simulink model "Drone_simulation_pilotage_en_vitesse_v5"  (R2016a)
settings: Solver=ode15s  StartTime=0.0  StopTime=6  FixedStep=0.01  MaxStep=0.01  RelTol=1e-3
undefined symbols (not defined in the file or in its folder): faut_sldprt, sigbuilder_block, sol_D, X, Y, Z
libraries: fl_lib x78, sm_lib x36, nesl_utility x15, simulink x1
(part 2 of 2)

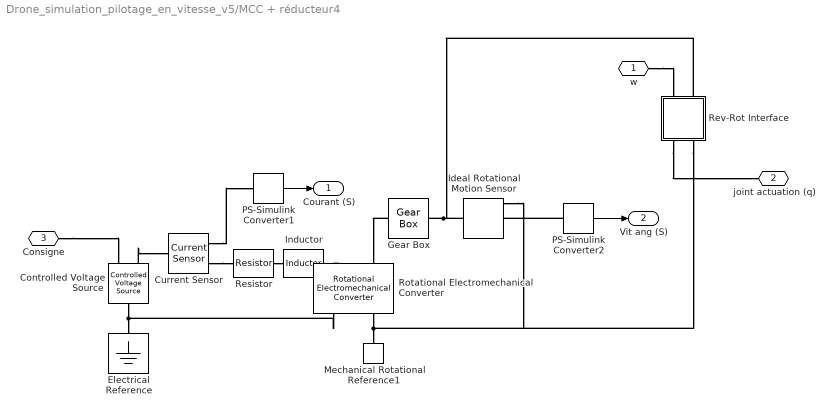
== system Drone_simulation_pilotage_en_vitesse_v5/MCC + réducteur4 ==
  Controlled Voltage Source : fl_lib/Electrical/Electrical Sources/Controlled Voltage Source
  Current Sensor : fl_lib/Electrical/Electrical Sensors/Current Sensor
  Electrical Reference : fl_lib/Electrical/Electrical Elements/Electrical Reference
  Gear Box : fl_lib/Mechanical/Mechanisms/Gear Box  ratio=6  t_in_specify=off  t_in_priority=High  t_in=0 N*m  t_out_specify=off  t_out_priority=High  t_out=0 N*m
  Ideal Rotational Motion Sensor : fl_lib/Mechanical/Mechanical Sensors/Ideal Rotational Motion Sensor  offset=0 rad
  Inductor : fl_lib/Electrical/Electrical Elements/Inductor  l=0.0003 H  r=0 Ohm  g=1e-9 1/Ohm  i_specify=off  i_priority=High  i=0 A  v_specify=off  v_priority=High  v=0 V  i_L_specify=off  i_L_priority=High  i_L=0 A
  Mechanical Rotational Reference1 : fl_lib/Mechanical/Rotational Elements/Mechanical Rotational Reference
  PS-Simulink Converter1 : nesl_utility/PS-Simulink Converter  PhysicalDomain=network_engine_domain  SubClassName=ps_output  LeftPortType=input  RightPortType=output  PseudoPeriodic=off  Frequencies=[]  Unit=1  AffineConversion=off
  PS-Simulink Converter2 : nesl_utility/PS-Simulink Converter  PhysicalDomain=network_engine_domain  SubClassName=ps_output  LeftPortType=input  RightPortType=output  PseudoPeriodic=off  Frequencies=[]  Unit=1  AffineConversion=off
  Resistor : fl_lib/Electrical/Electrical Elements/Resistor  R=2 Ohm  i_specify=off  i_priority=High  i=0 A  v_specify=off  v_priority=High  v=0 V
  Rev-Rot Interface : Subsystem
  Rotational Electromechanical Converter : fl_lib/Electrical/Electrical Elements/Rotational Electromechanical Converter  K=0.03 V/(rad/s)  i_specify=off  i_priority=High  i=0 A  v_specify=off  v_priority=High  v=0 V  t_specify=off  t_priority=High  t=0 N*m  w_specify=off  w_priority=High  w=0 rad/s
  w : PMIOPort  Port=1  Side=Left
  joint actuation (q) : PMIOPort  Port=2  Side=Left
  Consigne : PMIOPort  Port=3  Side=Left
  Courant (S) : Outport
  Vit ang (S) : Outport  Port=2
  wires:
  PS-Simulink Converter1/1 -> Courant (S)/1
  PS-Simulink Converter2/1 -> Vit ang (S)/1
  connections:
  Gear Box/LConn1 -- Rotational Electromechanical Converter/LConn2
  Controlled Voltage Source/RConn2 -- Current Sensor/LConn1
  Inductor/RConn1 -- Rotational Electromechanical Converter/LConn1
  Resistor/RConn1 -- Inductor/LConn1
  Current Sensor/RConn2 -- Resistor/LConn1
  Rotational Electromechanical Converter/RConn2 -- Mechanical Rotational Reference1/LConn1 -- Ideal Rotational Motion Sensor/RConn1 -- Rev-Rot Interface/LConn2
  PS-Simulink Converter2/LConn1 -- Ideal Rotational Motion Sensor/RConn2
  Rotational Electromechanical Converter/RConn1 -- Controlled Voltage Source/LConn1 -- Electrical Reference/LConn1
  Gear Box/RConn1 -- Ideal Rotational Motion Sensor/LConn1 -- Rev-Rot Interface/RConn2
  Current Sensor/RConn1 -- PS-Simulink Converter1/LConn1
  Consigne/RConn1 -- Controlled Voltage Source/RConn1
  w/RConn1 -- Rev-Rot Interface/RConn1
  Rev-Rot Interface/LConn1 -- joint actuation (q)/RConn1

== system Drone_simulation_pilotage_en_vitesse_v5/Signal Builder ==
  Demux : Demux  Tag=STV Demux  Outputs=1
  FromWs : FromWorkspace  Tag=STV FromWs  VariableName=tuvar  SampleTime=0
      SigBuilderData=|
      | common.afterFinalStr = 'Extrapolate'
      | common.sampleTime = 0
      | dataSet.timeRange = [0 10]
      | dataSet.name = 'Group 1'
      | sbobj.Groups.Name = 'Group 1'
      | sbobj.Groups.Signals.Name = 'Signal 1'
      | sbobj.Groups.Signals.XData = [0 1 3 4 5 10]
      | sbobj.Groups.Signals.YData = [0 0.5 0.5 0.2 0 0]
  Signal 1 : Outport  Tag=STV Outport
  wires:
  Demux/1 -> Signal 1/1
  FromWs/1 -> Demux/1

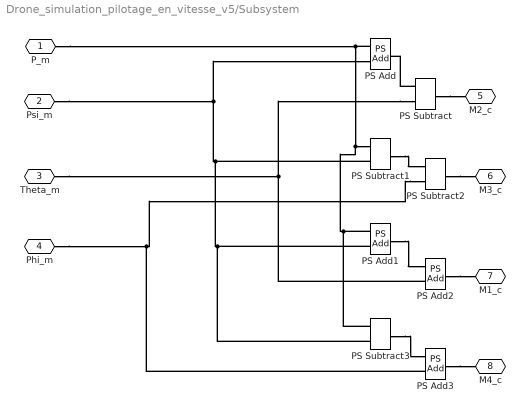
== system Drone_simulation_pilotage_en_vitesse_v5/Subsystem ==
  PS Add{,1..3} (4 alike) : fl_lib/Physical Signals/Functions/PS Add
  PS Subtract{,1..3} (4 alike) : fl_lib/Physical Signals/Functions/PS Subtract
  P_m : PMIOPort  Port=1  Side=Left
  Psi_m : PMIOPort  Port=2  Side=Left
  Theta_m : PMIOPort  Port=3  Side=Left
  Phi_m : PMIOPort  Port=4  Side=Left
  M2_c : PMIOPort  Port=5  Side=Right
  M3_c : PMIOPort  Port=6  Side=Right
  M1_c : PMIOPort  Port=7  Side=Right
  M4_c : PMIOPort  Port=8  Side=Right
  connections:
  PS Subtract1/RConn1 -- PS Subtract2/LConn1
  PS Subtract/LConn1 -- PS Add/RConn1
  PS Add/LConn2 -- Psi_m/RConn1 -- PS Subtract3/LConn2 -- PS Add1/LConn2 -- PS Subtract1/LConn2
  PS Add1/RConn1 -- PS Add2/LConn1
  PS Subtract2/LConn2 -- Phi_m/RConn1 -- PS Add3/LConn2
  PS Subtract/LConn2 -- Theta_m/RConn1 -- PS Add2/LConn2
  PS Subtract3/RConn1 -- PS Add3/LConn1
  PS Add/LConn1 -- PS Subtract3/LConn1 -- PS Add1/LConn1 -- PS Subtract1/LConn1 -- P_m/RConn1
  PS Add3/RConn1 -- M4_c/RConn1
  PS Add2/RConn1 -- M1_c/RConn1
  PS Subtract/RConn1 -- M2_c/RConn1
  PS Subtract2/RConn1 -- M3_c/RConn1

== system Drone_simulation_pilotage_en_vitesse_v5/sol_1_RIGID ==
  ReferenceFrame : sm_lib/Frames and Transforms/Reference Frame
  Solid : sm_lib/Body Elements/Solid  InertiaType=Custom  Mass=0.16  MassUnits=kg  CenterOfMass=[0 0 -0.5]  CenterOfMassUnits=mm  MomentsOfInertia=[2133.3466666666668 2133.3466666666668 4266.666666666667]  MomentsOfInertiaUnits=kg*mm^2  ProductsOfInertia=[0 0 0]  ProductsOfInertiaUnits=kg*mm^2  DensityBased=on  Density=1000  DensityUnits=kg/(m^3)  DoExposeReferenceFrame=on  SerializedFrames=<Frames/>  GraphicType=FromGeometry  MarkerShape=Sphere  MarkerSize=10  MarkerSizeUnits=m  GraphicVisPropType=SimpleVisualProperties  GraphicDiffuseColor=[0.79607843137254897 0.82352941176470584 0.93725490196078431]  GraphicSpecularColor=[0.5 0.5 0.5 1.0]  GraphicAmbientColor=[0.15 0.15 0.15 1.0]  GraphicEmissiveColor=[0.0 0.0 0.0 1.0]  GraphicShininess=75  GraphicOpacity=1  GeometryShape=FromFile  RectangleSize=[1 1]  RectangleSizeUnits=m  BrickDimensions=[1 1 1]  BrickDimensionUnits=m  CylinderRadius=1  CylinderRadiusUnits=m  CylinderLength=1  CylinderLengthUnits=m  SphereRadius=1  SphereRadiusUnits=m  EllipsoidRadii=[1 1 1]  EllipsoidRadiiUnits=m  ExtrusionCrossSection=[1 1; -1 1; -1 -1; 1 -1]  ExtrusionCrossSectionUnits=m  ExtrusionLength=1  ExtrusionLengthUnits=m  PolygonNumSides=3  PolygonOuterRadius=1  PolygonOuterRadiusUnits=m  ExtGeomFileType=STL  ExtGeomFileName=sol_D+®faut_sldprt.STL  ExtGeomFileUnits=mm  RevolutionCrossSection=[1 1; 1 -1; 2 -1; 2 1]  RevolutionCrossSectionUnits=m  RevolutionExtent=Full  RevolutionAngle=180  RevolutionAngleUnits=deg
  F : PMIOPort  Port=1  Side=Left
  connections:
  F/RConn1 -- ReferenceFrame/RConn1 -- Solid/RConn1

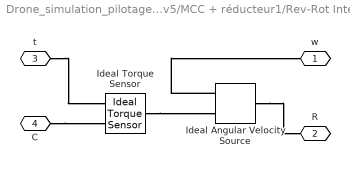
== system Drone_simulation_pilotage_en_vitesse_v5/MCC + réducteur1/Rev-Rot Interface ==
  Ideal Angular Velocity Source : fl_lib/Mechanical/Mechanical Sources/Ideal Angular Velocity Source
  Ideal Torque Sensor : fl_lib/Mechanical/Mechanical Sensors/Ideal Torque Sensor
  w : PMIOPort  Port=1  Side=Right
  R : PMIOPort  Port=2  Side=Right
  t : PMIOPort  Port=3  Side=Left
  C : PMIOPort  Port=4  Side=Left
  connections:
  Ideal Angular Velocity Source/RConn1 -- w/RConn1
  Ideal Torque Sensor/LConn1 -- Ideal Angular Velocity Source/RConn2
  C/RConn1 -- Ideal Torque Sensor/RConn1
  Ideal Angular Velocity Source/LConn1 -- R/RConn1
  t/RConn1 -- Ideal Torque Sensor/RConn2

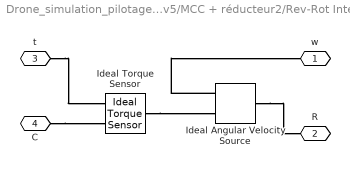
== system Drone_simulation_pilotage_en_vitesse_v5/MCC + réducteur2/Rev-Rot Interface ==
  Ideal Angular Velocity Source : fl_lib/Mechanical/Mechanical Sources/Ideal Angular Velocity Source
  Ideal Torque Sensor : fl_lib/Mechanical/Mechanical Sensors/Ideal Torque Sensor
  w : PMIOPort  Port=1  Side=Right
  R : PMIOPort  Port=2  Side=Right
  t : PMIOPort  Port=3  Side=Left
  C : PMIOPort  Port=4  Side=Left
  connections:
  Ideal Angular Velocity Source/RConn1 -- w/RConn1
  Ideal Torque Sensor/LConn1 -- Ideal Angular Velocity Source/RConn2
  C/RConn1 -- Ideal Torque Sensor/RConn1
  Ideal Angular Velocity Source/LConn1 -- R/RConn1
  t/RConn1 -- Ideal Torque Sensor/RConn2

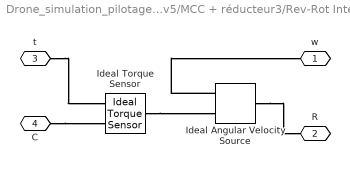
== system Drone_simulation_pilotage_en_vitesse_v5/MCC + réducteur3/Rev-Rot Interface ==
  Ideal Angular Velocity Source : fl_lib/Mechanical/Mechanical Sources/Ideal Angular Velocity Source
  Ideal Torque Sensor : fl_lib/Mechanical/Mechanical Sensors/Ideal Torque Sensor
  w : PMIOPort  Port=1  Side=Right
  R : PMIOPort  Port=2  Side=Right
  t : PMIOPort  Port=3  Side=Left
  C : PMIOPort  Port=4  Side=Left
  connections:
  Ideal Angular Velocity Source/RConn1 -- w/RConn1
  Ideal Torque Sensor/LConn1 -- Ideal Angular Velocity Source/RConn2
  C/RConn1 -- Ideal Torque Sensor/RConn1
  Ideal Angular Velocity Source/LConn1 -- R/RConn1
  t/RConn1 -- Ideal Torque Sensor/RConn2

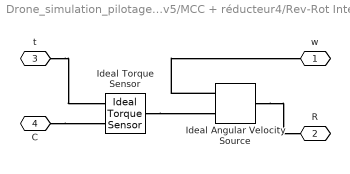
== system Drone_simulation_pilotage_en_vitesse_v5/MCC + réducteur4/Rev-Rot Interface ==
  Ideal Angular Velocity Source : fl_lib/Mechanical/Mechanical Sources/Ideal Angular Velocity Source
  Ideal Torque Sensor : fl_lib/Mechanical/Mechanical Sensors/Ideal Torque Sensor
  w : PMIOPort  Port=1  Side=Right
  R : PMIOPort  Port=2  Side=Right
  t : PMIOPort  Port=3  Side=Left
  C : PMIOPort  Port=4  Side=Left
  connections:
  Ideal Angular Velocity Source/RConn1 -- w/RConn1
  Ideal Torque Sensor/LConn1 -- Ideal Angular Velocity Source/RConn2
  C/RConn1 -- Ideal Torque Sensor/RConn1
  Ideal Angular Velocity Source/LConn1 -- R/RConn1
  t/RConn1 -- Ideal Torque Sensor/RConn2
